simulink model "adc_demo"  (R2023a)
settings: Solver=VariableStepDiscrete  StartTime=0.0  StopTime=1  RelTol=1e-3  EnableMultiTasking=on
libraries: simulink_extras x1
settings Model: Creator=rcheng  LastModifiedBy=Juan
settings SolverCC: AlgebraicLoopSolver=TrustRegion
settings DataIOCC: LimitDataPoints=on  SaveFormat=Array  SignalLoggingSaveFormat=ModelDataLogs  ReturnWorkspaceOutputs=off
settings OptimizationCC: ExpressionDepthLimit=2147483647  InitFltsAndDblsToZero=on  LifeSpan=inf
settings DebuggingCC: UnderspecifiedInitializationDetection=Classic  MergeDetectMultiDrivingBlocksExec=none  SolverPrmCheckMsg=warning  FcnCallInpInsideContextMsg=warning  UnconnectedInputMsg=warning  UnconnectedOutputMsg=warning  UnconnectedLineMsg=warning  StateNameClashWarn=warning  SFUnexpectedBacktrackingDiag=warning  SFNoUnconditionalDefaultTransitionDiag=warning  SFExecutionAtInitializationDiag=none  ArithmeticOperatorsInVariantConditions=warning
settings HardwareCC: ProdBitPerPointer=32  ProdBitPerSizeT=32  ProdBitPerPtrDiffT=32  ProdLargestAtomicFloat=None  ProdIntDivRoundTo=Undefined  ProdEndianess=Unspecified  ProdWordSize=32  ProdHWDeviceType=32-bit Generic
settings ModelReferenceCC: EnableRefExpFcnMdlSchedulingChecks=on  PropagateSignalLabelsOutOfModel=off
settings SFSimCC: SimUseLocalCustomCode=off  CustomCodeUndefinedFunction=UseInterfaceOnly
settings RTWCC: RTWUseLocalCustomCode=off  DLArmComputeVersion=19.05
settings CodeAppCC: StateflowObjectComments=on
settings GRTTargetCC: TargetLangStandard=C89/C90 (ANSI)  CombineOutputUpdateFcns=off  GRTInterface=on
settings ConfigComp: CovMetricSettings=dw  CovSaveCumulativeToWorkspaceVar=on  CovSaveSingleToWorkspaceVar=on  CovExternalEMLEnable=off  CovSFcnEnable=off

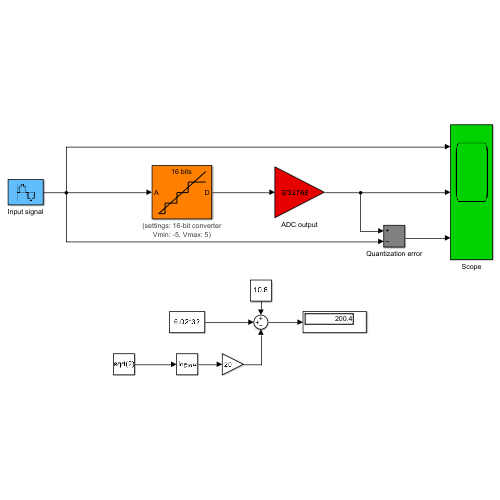
[thumbnail: Simulink's stored preview of the top-level diagram]
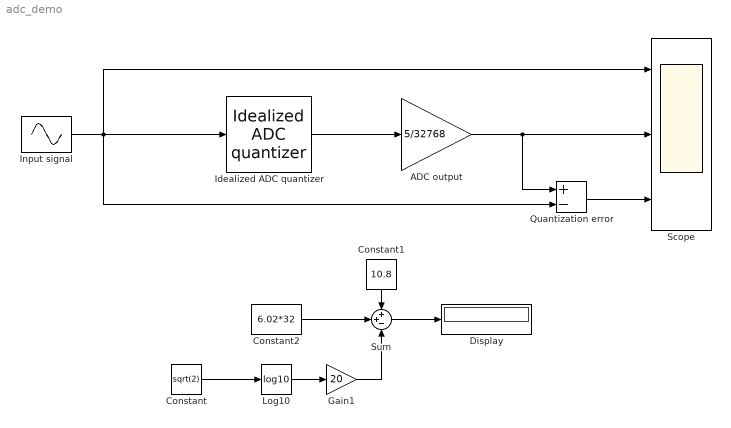
== system adc_demo ==
  ADC output : Gain  Gain=5/32768
  Constant : Constant  Value=sqrt(2)
  Constant1 : Constant  Value=10.8
  Constant2 : Constant  Value=6.02*32
  Display : Display
  Gain1 : Gain  Gain=20
  Idealized ADC quantizer : simulink_extras/Additional Discrete/Idealized ADC quantizer  NumberOfConverterBits=16  Vmin=-5  Vmax=5  OutputDataType=int16  OutputNegativeValues=on
  Input signal : Sin  Amplitude=2.5  Frequency=2*pi*100  SampleTime=1/10000
  Log10 : Math  Operator=log10
  Quantization error : Sum  Inputs=+-
  Scope : Scope  NumInputPorts=3
  Sum : Sum  Inputs=++-
  wires:
  Idealized ADC quantizer/1 -> ADC output/1
  ADC output/1 -> Quantization error/1, Scope/2
  Input signal/1 -> Idealized ADC quantizer/1, Quantization error/2, Scope/1
  Quantization error/1 -> Scope/3
  Constant/1 -> Log10/1
  Log10/1 -> Gain1/1
  Gain1/1 -> Sum/3
  Constant2/1 -> Sum/2
  Constant1/1 -> Sum/1
  Sum/1 -> Display/1
